simulink model "Pacemaker"  (R2022b)
settings: Solver=FixedStepAuto  StartTime=0.0  StopTime=10.0  FixedStep=1e-3  RelTol=1e-3  EnableMultiTasking=on
undefined symbols (not defined in the file): D0, D1, D10, D11, D12, D13, D2, D3, D4, D5, D6, D7, D8, D9, PTA0, PTA1, PTA2, PTB23, PTB9, PTC16, PTC17, PTC2, PTC3, PTC4, PTD0, PTD1, PTD2, PTD3
libraries: frdmk64flib x14
settings Model: ExtModeTrigDuration=5  Creator=ecmce  LastModifiedBy=ecmce
settings OptimizationCC: EnhancedBackFolding=on  PassReuseOutputArgsAs=Individual arguments  ZeroExternalMemoryAtStartup=off  ZeroInternalMemoryAtStartup=off  MaxStackSize=64  OptimizeBlockOrder=speed  DifferentSizesBufferReuse=on  OptimizationCustomize=off  EfficientTunableParamExpr=on
settings DebuggingCC: ParameterTunabilityLossMsg=error
settings HardwareCC: ProdBitPerPointer=32  ProdBitPerSizeT=32  ProdBitPerPtrDiffT=32  ProdLargestAtomicInteger=Long  ProdLargestAtomicFloat=Double  ProdWordSize=32  ProdHWDeviceType=ARM Compatible->ARM Cortex
settings SFSimCC: MATLABDynamicMemAlloc=off
settings RTWCC: Description=Embedded Coder  SystemTargetFile=ert.tlc  HardwareBoard=NXP FRDM-K64F  TLCOptions="-aInlineSetEventsForThisBaseRateFcn=TLC_FALSE -aSuppressMultiTaskScheduler=TLC_FALSE  -aRateBasedStepFcn=0"  TemplateMakefile=ert_default_tmf  Toolchain=GNU Tools for ARM Embedded Processors
settings CodeAppCC: ForceParamTrailComments=on  IgnoreCustomStorageClasses=off  OperatorAnnotations=on  SimulinkDataObjDesc=on  SFDataObjDesc=on  InsertBlockDesc=on
settings ERTTargetCC: ExtModeTransport=4  ExtModeMexFile=sendToCommService

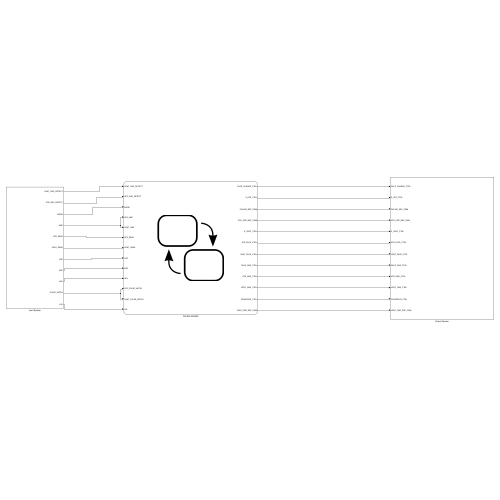
[thumbnail: Simulink's stored preview of the top-level diagram]
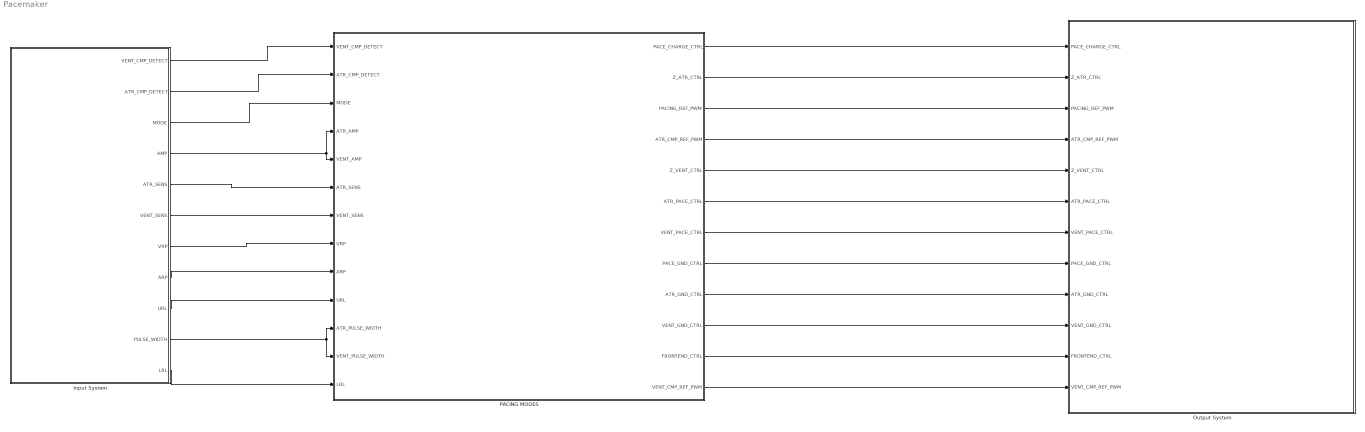
== system Pacemaker ==
  Input System : Subsystem
  Output System : Subsystem
  PACING MODES : Stateflow chart  TreatAsAtomicUnit=on
      settings: PortSchema="{\"entries\":[{\"content\":{\"sides\":[{\"content\":{\"connectorIds\":[\"In1\",\"In2\",\"In12\",\"In4\",\"In6\",\"In9\",\"In13\",\"In10\",\"In11\",\"In5\",\"In7\",\"In8\",\"In3\"]},\"type\":\"ConnectorPlacement.EquallySpacedRectSide\",\"uuid\":\"b9290718-055f-4c31-bc3d-b0976e8c48fd\"},{\"content\":{\"connectorIds\":[\"Out1\",\"Out2\",\"Out3\",\"Out4\",\"Out5\",\"Out6\",\"Out7\",\"Out8\",\"Out9\",\"Out10\",\"Out11\",\"Out12\"],\"side\":\"RIGHT\"},\"type\":\"ConnectorPlacement.EquallySpacedRectSide\",\"uuid\":\"0535c7c4-5dc5-4080-8ff5-112da28c2564\"},{\"content\":{\"connectorIds\":[],\"side\":\"TOP\"},\"type\":\"ConnectorPlacement.EquallySpacedRectSide\",\"uuid\":\"4d7cc439-c207-4c97-8163-52fd6fc810bf\"}]},\"type\":\"ConnectorPlacement.EquallySpacedConnector\",\"uuid\":\"b748d944-c975-4847-b57b-75350a5981d6\"}],\"packageUris\":[\"http://schema.mathworks.com/mf0/Connector/R2020b\"],\"version\":\"1.0\"}"
  wires:
  PACING MODES/1(PACE_CHARGE_CTRL) -> Output System/1(PACE_CHARGE_CTRL)
  PACING MODES/2(Z_ATR_CTRL) -> Output System/2(Z_ATR_CTRL)
  PACING MODES/3(PACING_REF_PWM) -> Output System/3(PACING_REF_PWM)
  PACING MODES/4(ATR_CMP_REF_PWM) -> Output System/4(ATR_CMP_REF_PWM)
  PACING MODES/5(Z_VENT_CTRL) -> Output System/5(Z_VENT_CTRL)
  PACING MODES/6(ATR_PACE_CTRL) -> Output System/6(ATR_PACE_CTRL)
  PACING MODES/7(VENT_PACE_CTRL) -> Output System/7(VENT_PACE_CTRL)
  PACING MODES/8(PACE_GND_CTRL) -> Output System/8(PACE_GND_CTRL)
  PACING MODES/9(ATR_GND_CTRL) -> Output System/9(ATR_GND_CTRL)
  PACING MODES/10(VENT_GND_CTRL) -> Output System/10(VENT_GND_CTRL)
  PACING MODES/11(FRONTEND_CTRL) -> Output System/11(FRONTEND_CTRL)
  PACING MODES/12(VENT_CMP_REF_PWM) -> Output System/12(VENT_CMP_REF_PWM)
  Input System/1(VENT_CMP_DETECT) -> PACING MODES/1(VENT_CMP_DETECT)
  Input System/2(ATR_CMP_DETECT) -> PACING MODES/2(ATR_CMP_DETECT)
  Input System/3(MODE) -> PACING MODES/12(MODE)
  Input System/9(URL) -> PACING MODES/5(URL)
  Input System/4(AMP) -> PACING MODES/6(VENT_AMP), PACING MODES/4(ATR_AMP)
  Input System/7(VRP) -> PACING MODES/10(VRP)
  Input System/8(ARP) -> PACING MODES/11(ARP)
  Input System/6(VENT_SENS) -> PACING MODES/13(VENT_SENS)
  Input System/10(PULSE_WIDTH) -> PACING MODES/8(VENT_PULSE_WIDTH), PACING MODES/7(ATR_PULSE_WIDTH)
  Input System/5(ATR_SENS) -> PACING MODES/9(ATR_SENS)
  Input System/11(LRL) -> PACING MODES/3(LRL)

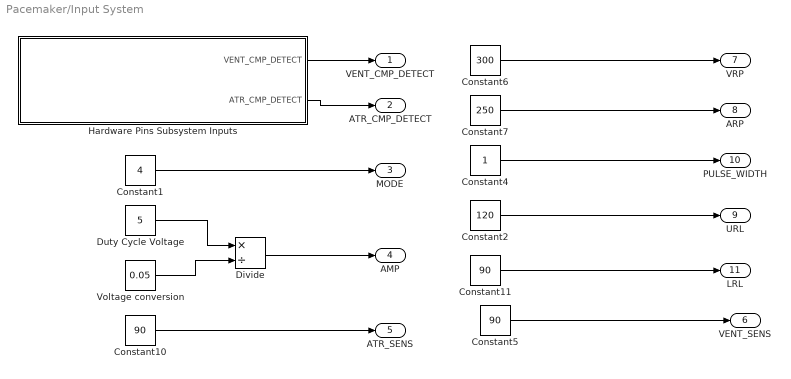
== system Pacemaker/Input System ==
  Constant1 : Constant  Value=4
  Constant10 : Constant  Value=90
  Constant11 : Constant  Value=90
  Constant2 : Constant  Value=120
  Constant4 : Constant
  Constant5 : Constant  Value=90
  Constant6 : Constant  Value=300
  Constant7 : Constant  Value=250
  Divide : Product  Inputs=*/
  Duty Cycle Voltage : Constant  Value=5
  Hardware Pins Subsystem Inputs : Subsystem
  Voltage conversion : Constant  Value=0.05
  VENT_CMP_DETECT : Outport
  ATR_CMP_DETECT : Outport  Port=2
  MODE : Outport  Port=3
  AMP : Outport  Port=4
  ATR_SENS : Outport  Port=5
  VENT_SENS : Outport  Port=6
  VRP : Outport  Port=7
  ARP : Outport  Port=8
  URL : Outport  Port=9
  PULSE_WIDTH : Outport  Port=10
  LRL : Outport  Port=11
  wires:
  Constant7/1 -> ARP/1
  Constant6/1 -> VRP/1
  Constant11/1 -> LRL/1
  Constant2/1 -> URL/1
  Hardware Pins Subsystem Inputs/2(ATR_CMP_DETECT) -> ATR_CMP_DETECT/1
  Constant5/1 -> VENT_SENS/1
  Constant10/1 -> ATR_SENS/1
  Constant1/1 -> MODE/1
  Hardware Pins Subsystem Inputs/1(VENT_CMP_DETECT) -> VENT_CMP_DETECT/1
  Constant4/1 -> PULSE_WIDTH/1
  Duty Cycle Voltage/1 -> Divide/1
  Divide/1 -> AMP/1
  Voltage conversion/1 -> Divide/2

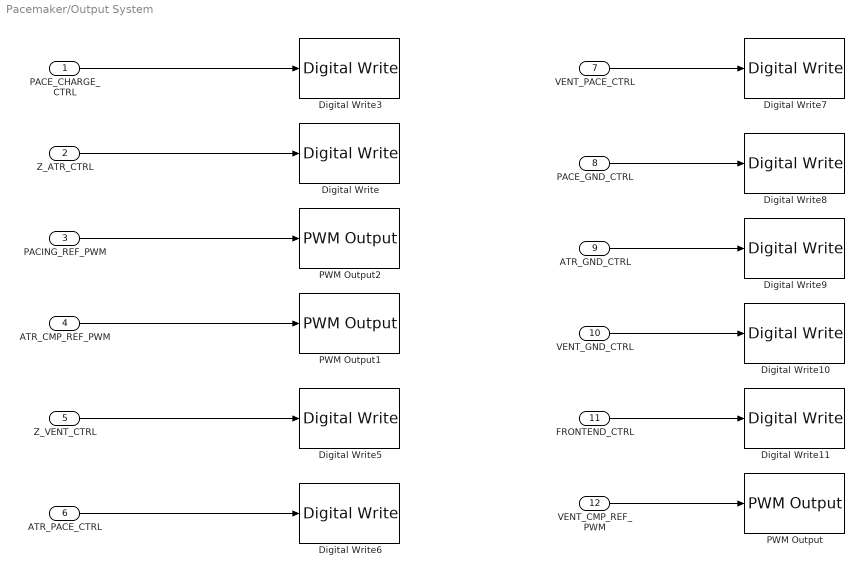
== system Pacemaker/Output System ==
  PACE_CHARGE_CTRL : Inport  OutDataTypeStr=boolean
  Z_ATR_CTRL : Inport  Port=2  OutDataTypeStr=boolean
  PACING_REF_PWM : Inport  Port=3  OutDataTypeStr=double
  ATR_CMP_REF_PWM : Inport  Port=4  OutDataTypeStr=double
  Z_VENT_CTRL : Inport  Port=5  OutDataTypeStr=boolean
  ATR_PACE_CTRL : Inport  Port=6  OutDataTypeStr=boolean
  VENT_PACE_CTRL : Inport  Port=7  OutDataTypeStr=boolean
  PACE_GND_CTRL : Inport  Port=8  OutDataTypeStr=boolean
  ATR_GND_CTRL : Inport  Port=9  OutDataTypeStr=boolean
  VENT_GND_CTRL : Inport  Port=10  OutDataTypeStr=boolean
  FRONTEND_CTRL : Inport  Port=11  OutDataTypeStr=boolean
  VENT_CMP_REF_PWM : Inport  Port=12  OutDataTypeStr=double
  Digital Write : frdmk64flib/Digital Write  Whichpin=PTB23 (D4)
  Digital Write10 : frdmk64flib/Digital Write  Whichpin=PTD3 (D12)
  Digital Write11 : frdmk64flib/Digital Write  Whichpin=PTD1 (D13)
  Digital Write3 : frdmk64flib/Digital Write  Whichpin=PTB9 (D2)
  Digital Write5 : frdmk64flib/Digital Write  Whichpin=PTC3 (D7)
  Digital Write6 : frdmk64flib/Digital Write  Whichpin=PTA0 (D8)
  Digital Write7 : frdmk64flib/Digital Write  Whichpin=PTC4 (D9)
  Digital Write8 : frdmk64flib/Digital Write  Whichpin=PTD0 (D10)
  Digital Write9 : frdmk64flib/Digital Write  Whichpin=PTD2 (D11)
  PWM Output : frdmk64flib/PWM Output  Whichpin=PTA1 (D3)  InitialFrequency=2000  InitialDutyCycle=0
  PWM Output1 : frdmk64flib/PWM Output  Whichpin=PTC2 (D6)  InitialFrequency=2000  InitialDutyCycle=0
  PWM Output2 : frdmk64flib/PWM Output  Whichpin=PTA2 (D5)  InitialFrequency=2000  InitialDutyCycle=0
  wires:
  Z_ATR_CTRL/1 -> Digital Write/1
  PACING_REF_PWM/1 -> PWM Output2/1
  PACE_CHARGE_CTRL/1 -> Digital Write3/1
  ATR_CMP_REF_PWM/1 -> PWM Output1/1
  VENT_CMP_REF_PWM/1 -> PWM Output/1
  Z_VENT_CTRL/1 -> Digital Write5/1
  ATR_PACE_CTRL/1 -> Digital Write6/1
  VENT_PACE_CTRL/1 -> Digital Write7/1
  PACE_GND_CTRL/1 -> Digital Write8/1
  ATR_GND_CTRL/1 -> Digital Write9/1
  VENT_GND_CTRL/1 -> Digital Write10/1
  FRONTEND_CTRL/1 -> Digital Write11/1

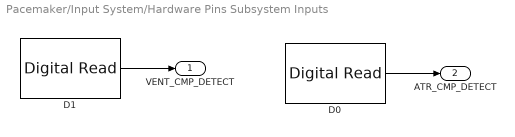
== system Pacemaker/Input System/Hardware Pins Subsystem Inputs ==
  D0 : frdmk64flib/Digital Read  Whichpin=PTC16 (D0)  SampleTime=-1
  D1 : frdmk64flib/Digital Read  Whichpin=PTC17 (D1)  SampleTime=-1
  VENT_CMP_DETECT : Outport
  ATR_CMP_DETECT : Outport  Port=2
  wires:
  D1/1 -> VENT_CMP_DETECT/1
  D0/1 -> ATR_CMP_DETECT/1

== stateflow chart Pacemaker/PACING MODES ==
  state INIT
    entry:
    % set parameters to false initially
    VENT_PACE_CTRL = false;
    PACE_GND_CTRL = false;
    ATR_GND_CTRL = false;
    ATR_PACE_CTRL = false;
    VENT_GND_CTRL = false;
  state AOO
    state AOO_PACING
      %Discharging C22 and charging C21
      entry:
      % Set control signals for atrial pacing
      PACE_CHARGE_CTRL = false; %disable charging
      PACE_GND_CTRL = true; %enable ground control for pacing (Safety)
      ATR_PACE_CTRL = true; %enables atrial pacing
      ATR_GND_CTRL = false; %disable ground control for atrial
      %impedance monitoring is not necessary so it is disabled
      Z_ATR_CTRL = false; %disable impedance monitoring for atrial
      Z_VENT_CTRL = false; %disable impedance monitoring for ventrical
    state AOO_CHARGE
      %charge C22 and discharging C21
      entry:
      % Set control signals for charging
      PACE_GND_CTRL = true; %ground control enabled for pacing (for safety)
      ATR_PACE_CTRL = false; %Disable atrial pacing while charging
      PACING_REF_PWM = ATR_AMP;
      PACE_CHARGE_CTRL = true; %enable charging for C22
      %enable
      ATR_GND_CTRL = true; %enable ground (safety) in atrium while charging
    (default) -> AOO_CHARGE
    AOO_CHARGE -> AOO_PACING : [after(60000/LRL - ATR_PULSE_WIDTH, msec)]%time delay after charginng the pacemaker
    AOO_PACING -> AOO_CHARGE : after(ATR_PULSE_WIDTH,msec)
  state VVI
    state VVI_CHARGE
      entry:
      %charging C22
      FRONTEND_CTRL = false;
      VENT_PACE_CTRL = false;
      %ATR and VENT _PACE_CTRL must be off to avoid connecting patient directly to PWM
      PACING_REF_PWM = VENT_AMP;
      PACE_CHARGE_CTRL = true;
      VENT_CMP_REF_PWM = VENT_SENS;
      %discharging C21
      PACE_GND_CTRL = true; %allows charge to accumulate in C21
      Z_ATR_CTRL = false;
      Z_VENT_CTRL = false;
      VENT_GND_CTRL = true;
    state VVI_PACING
      entry:
      PACE_CHARGE_CTRL = false;
      PACE_GND_CTRL = true;
      Z_ATR_CTRL = false;
      Z_VENT_CTRL = false;
      VENT_GND_CTRL = false;
      VENT_PACE_CTRL = true;
    state VVI_REFACTORY
      entry:
      FRONTEND_CTRL = true;
    (default) -> VVI_CHARGE
    VVI_PACING -> VVI_CHARGE : after(VENT_PULSE_WIDTH,msec)
    VVI_REFACTORY -> VVI_PACING [order 1] : [(VENT_CMP_DETECT == 0) && after(60000/LRL-VRP-VENT_PULSE_WIDTH,msec)]
    VVI_REFACTORY -> VVI_CHARGE [order 2] : [(VENT_CMP_DETECT == 1)]
    VVI_CHARGE -> VVI_REFACTORY : [after(VRP,msec)]
  state MODE_SELECT
    entry:
    % based on mode go to pacing mode
  state VOO
    state VOO_Charge
      entry:
      ATR_PACE_CTRL = false;
      VENT_PACE_CTRL = false;
      PACING_REF_PWM = VENT_AMP;
      PACE_CHARGE_CTRL = true;
      %
      PACE_GND_CTRL = true;
      Z_ATR_CTRL = false;
      Z_VENT_CTRL = false;
      ATR_GND_CTRL = false;
      VENT_GND_CTRL = true;
    state VOO_Pace
      entry:
      PACE_CHARGE_CTRL = false;
      PACE_GND_CTRL = true;
      ATR_PACE_CTRL = false;
      ATR_GND_CTRL = false;
      Z_ATR_CTRL = false;
      Z_VENT_CTRL = false;
      VENT_GND_CTRL = false;
      VENT_PACE_CTRL = true;
    (default) -> VOO_Charge
    VOO_Pace -> VOO_Charge : [after(ATR_PULSE_WIDTH, msec)]
    VOO_Charge -> VOO_Pace : [after(60000/LRL - VENT_PULSE_WIDTH, msec)]%after charging
  state AAI
    state AAI_CHARGE
      %charge C22
      entry:
      FRONTEND_CTRL = false;
      ATR_PACE_CTRL = false;
      PACING_REF_PWM = ATR_AMP;
      PACE_CHARGE_CTRL = true;
      ATR_CMP_REF_PWM = ATR_SENS;
      %discharge C21
      PACE_GND_CTRL = true;
      Z_ATR_CTRL = false;
      Z_VENT_CTRL = false;
      ATR_GND_CTRL = true;
      %ATR_PACE_CTRL = false;
    state AAI_PACING
      entry:
      PACE_CHARGE_CTRL = false;
      PACE_GND_CTRL = true;
      ATR_PACE_CTRL = true;
      ATR_GND_CTRL = false;
      Z_ATR_CTRL = false;
      Z_VENT_CTRL = false;
    state AAI_REFRACTORY
      entry:
      %charged and ready to deliver pace.
      %wait refractory period then deliver pace
      %or return to charging state depending
      %on if a rythym is detected.
      FRONTEND_CTRL = true;
    (default) -> AAI_CHARGE
    AAI_PACING -> AAI_CHARGE : [after(ATR_PULSE_WIDTH, msec)]
    AAI_REFRACTORY -> AAI_CHARGE [order 1] : [ATR_CMP_DETECT==1]
        | % Pulse detected -do not pace
    AAI_CHARGE -> AAI_REFRACTORY : [after(ARP,msec)]
    AAI_REFRACTORY -> AAI_PACING [order 2] : [ATR_CMP_DETECT == 0 && after(60000/LRL-ARP- ATR_PULSE_WIDTH, msec)]
        | %no pulse detected - pacing necessary
  (default) -> INIT
  INIT -> MODE_SELECT : [after(100,msec)]
  MODE_SELECT -> AOO [order 2] : [MODE == 1]
  MODE_SELECT -> VVI [order 4] : [MODE == 4]
  MODE_SELECT -> VOO [order 3] : [MODE == 2]
  MODE_SELECT -> AAI [order 1] : [MODE == 3]
  data: PACE_CHARGE_CTRL output boolean size=1; Z_ATR_CTRL output boolean size=1; PACING_REF_PWM output double size=1; ATR_CMP_REF_PWM output double size=1; Z_VENT_CTRL output boolean size=1; ATR_PACE_CTRL output boolean size=1; VENT_PACE_CTRL output boolean size=1; PACE_GND_CTRL output boolean size=1; ATR_GND_CTRL output boolean size=1; VENT_GND_CTRL output boolean size=1; FRONTEND_CTRL output boolean size=1; VENT_CMP_DETECT input boolean size=1; ATR_CMP_DETECT input boolean size=1; LRL input double size=1; ATR_AMP input double size=1; URL input double size=1; VENT_AMP input double size=1; ATR_PULSE_WIDTH input double size=1; VENT_PULSE_WIDTH input double size=1; ATR_SENS input double size=1; VRP input double size=1; ARP input double size=1; MODE input double size=1; VENT_CMP_REF_PWM output double size=1; VENT_SENS input double size=1
